simulink model "capitol4pb3"  (R2013a)
settings: Solver=ode45  StartTime=0.0  StopTime=14400  RelTol=1e-3
undefined symbols (not defined in the file): des, gcbh
settings Model: Creator=user  LastModifiedBy=user

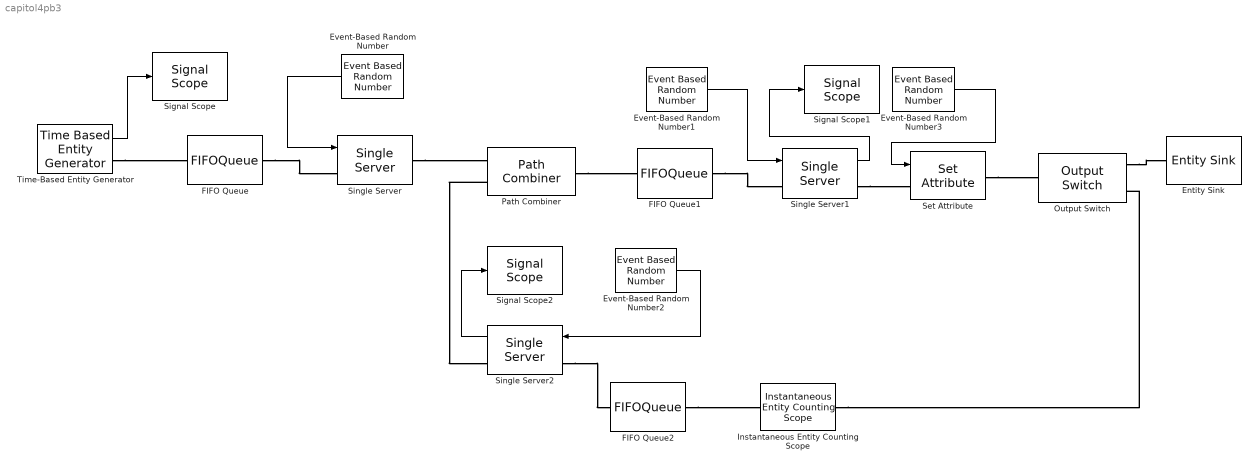
== system capitol4pb3 ==
  Entity Sink : EntitySink
  Event-Based Random Number : EventBasedRandomNumber  Distribution=Uniform  minUnif=40  maxUnif=80
  Event-Based Random Number1 : EventBasedRandomNumber  Distribution=Uniform  minUnif=120  maxUnif=240
  Event-Based Random Number2 : EventBasedRandomNumber  Distribution=Uniform  minUnif=70  maxUnif=170
  Event-Based Random Number3 : EventBasedRandomNumber  Distribution=Arbitrary discrete  valueVecDisc=[1 2]  probVecDisc=[0.70 0.30]
  FIFO Queue : FIFOQueue
  FIFO Queue1 : FIFOQueue
  FIFO Queue2 : FIFOQueue
  Instantaneous Entity Counting Scope : InstantaneousEntityCountingScope  LoadFcn=des.scope.CallbackSupport('seLoadFcn',gcbh)  StartFcn=des.scope.CallbackSupport('seStartFcn',gcbh)  StopFcn=des.scope.CallbackSupport('seStopFcn',gcbh)
      settings: CopyFcn=des.scope.CallbackSupport('seCopyFcn',gcbh)  DeleteFcn=des.scope.CallbackSupport('seDeleteFcn',gcbh)  PreSaveFcn=des.scope.CallbackSupport('sePreSaveFcn',gcbh)  NameChangeFcn=des.scope.CallbackSupport('seNameChangeFcn',gcbh)  OpenFcn=des.scope.CallbackSupport('seOpenFcn',gcbh)
  Output Switch : OutputSwitch  NumberOutputPorts=2  SwitchingCriterion=From attribute  AttributeName=TestPassed
  Path Combiner : PathCombiner  NumberInputPorts=2
  Set Attribute : SetAttribute  AttributeName=Attribute1|TestPassed  AttributeFrom=Dialog|Signal port  AttributeValue=1|1  AttributeTreatAsVector=1|1  EvaluatedAttributeValue={ 1;[]}
      settings: InputPortMap=u1
  Signal Scope : SignalScope  LoadFcn=des.scope.CallbackSupport('seLoadFcn',gcbh)  StartFcn=des.scope.CallbackSupport('seStartFcn',gcbh)  StopFcn=des.scope.CallbackSupport('seStopFcn',gcbh)
      settings: CopyFcn=des.scope.CallbackSupport('seCopyFcn',gcbh)  DeleteFcn=des.scope.CallbackSupport('seDeleteFcn',gcbh)  PreSaveFcn=des.scope.CallbackSupport('sePreSaveFcn',gcbh)  NameChangeFcn=des.scope.CallbackSupport('seNameChangeFcn',gcbh)  OpenFcn=des.scope.CallbackSupport('seOpenFcn',gcbh)
  Signal Scope1 : SignalScope  LoadFcn=des.scope.CallbackSupport('seLoadFcn',gcbh)  StartFcn=des.scope.CallbackSupport('seStartFcn',gcbh)  StopFcn=des.scope.CallbackSupport('seStopFcn',gcbh)
      settings: CopyFcn=des.scope.CallbackSupport('seCopyFcn',gcbh)  DeleteFcn=des.scope.CallbackSupport('seDeleteFcn',gcbh)  PreSaveFcn=des.scope.CallbackSupport('sePreSaveFcn',gcbh)  NameChangeFcn=des.scope.CallbackSupport('seNameChangeFcn',gcbh)  OpenFcn=des.scope.CallbackSupport('seOpenFcn',gcbh)
  Signal Scope2 : SignalScope  LoadFcn=des.scope.CallbackSupport('seLoadFcn',gcbh)  StartFcn=des.scope.CallbackSupport('seStartFcn',gcbh)  StopFcn=des.scope.CallbackSupport('seStopFcn',gcbh)
      settings: CopyFcn=des.scope.CallbackSupport('seCopyFcn',gcbh)  DeleteFcn=des.scope.CallbackSupport('seDeleteFcn',gcbh)  PreSaveFcn=des.scope.CallbackSupport('sePreSaveFcn',gcbh)  NameChangeFcn=des.scope.CallbackSupport('seNameChangeFcn',gcbh)  OpenFcn=des.scope.CallbackSupport('seOpenFcn',gcbh)
  Single Server : SingleServer  ServiceTimeFrom=Signal port t
  Single Server1 : SingleServer  ServiceTimeFrom=Signal port t  StatNumberDeparted=on
  Single Server2 : SingleServer  ServiceTimeFrom=Signal port t  StatNumberDeparted=on
  Time-Based Entity Generator : TimeBasedEntityGenerator  Distribution=Uniform  Period=0.5  Minimum=60  Maximum=180  StatNumberDeparted=on
  wires:
  Time-Based Entity Generator/1 -> Signal Scope/1
  Event-Based Random Number/1 -> Single Server/1
  Event-Based Random Number1/1 -> Single Server1/1
  Single Server1/1 -> Signal Scope1/1
  Single Server2/1 -> Signal Scope2/1
  Event-Based Random Number2/1 -> Single Server2/1
  Event-Based Random Number3/1 -> Set Attribute/1
  connections:
  Time-Based Entity Generator/RConn1 -- FIFO Queue/LConn1
  FIFO Queue/RConn1 -- Single Server/LConn1
  Single Server/RConn1 -- Path Combiner/LConn1
  Path Combiner/RConn1 -- FIFO Queue1/LConn1
  FIFO Queue1/RConn1 -- Single Server1/LConn1
  Single Server1/RConn1 -- Set Attribute/LConn1
  Set Attribute/RConn1 -- Output Switch/LConn1
  Output Switch/RConn1 -- Entity Sink/LConn1
  Path Combiner/LConn2 -- Single Server2/RConn1
  Single Server2/LConn1 -- FIFO Queue2/RConn1
  FIFO Queue2/LConn1 -- Instantaneous Entity Counting Scope/RConn1
  Instantaneous Entity Counting Scope/LConn1 -- Output Switch/RConn2
